simulink subsystem "drive"  (R2022a)
settings: Solver=VariableStepAuto  StartTime=0.0  StopTime=10.0  RelTol=1e-3
settings Model: Creator=12191  LastModifiedBy=12191

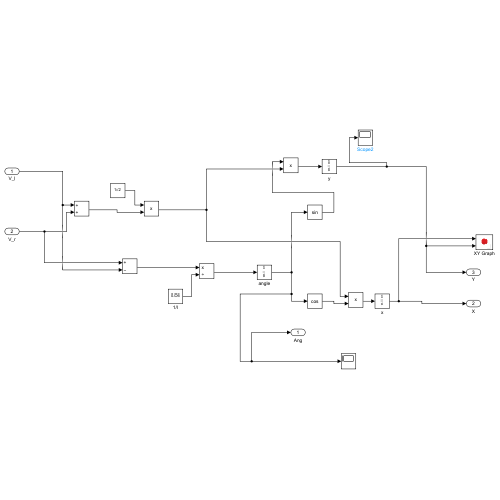
[thumbnail: Simulink's stored preview of the top-level diagram]
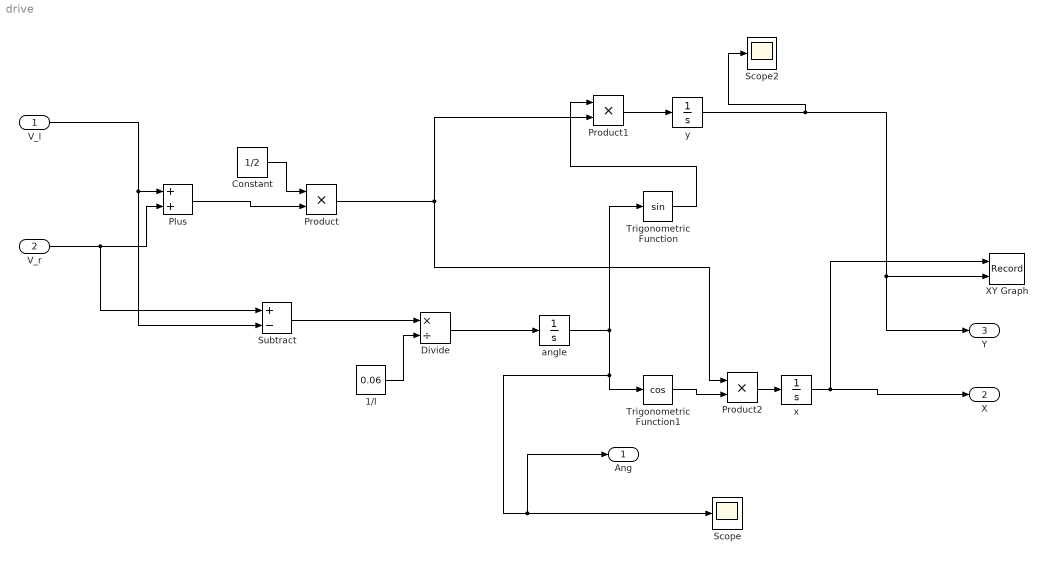
== system drive ==
  V_l : Inport
  V_r : Inport  Port=2
  1/l : Constant  Value=0.06
  Constant : Constant  Value=1/2
  Divide : Product  Inputs=*/
  Plus : Sum
  Product : Product
  Product1 : Product
  Product2 : Product
  Scope : Scope
  Scope2 : Scope
  Subtract : Sum  Inputs=+-
  Trigonometric Function : Trigonometry
  Trigonometric Function1 : Trigonometry  Operator=cos
  XY Graph : Record  FileSettingsInternal="{\"entries\":[{\"content\":{\"excelSettings\":{\"content\":{},\"type\":\"Streamout.ExcelSettings\"}},\"type\":\"Streamout.FileSettingStorage\",\"uuid\":\"175092fb-4bae-40dd-9490-6dec79859699\"}],\"packageUris\":[\"http://schema.mathworks.com/mf0/streamout_blocks/R2020a\"],\"version\":\"1.0\"}"  Layout=[1 1]  SignalsInternal="{\"entries\":[{\"content\":{\"signals\":[{\"content\":{\"blockPath\":[\"drive/XY Graph\"],\"channel\":[],\"dimensions\":[1],\"domain\":\"drive/XY Graph\",\"lineColor\":\"#a2142f\",\"plots\":[],\"port\":1,\"sid\":[],\"signalID\":747,\"signalName\":\"angle2\"},\"type\":\"RecordBlkView.Signal\",\"uuid\":\"ca3ea469-2ea0-4ac0-a534-a51894ec1fa5\"},{\"content\":{\"blockPath\":[\"drive/XY Graph\"],\"channel\":[],\"dimensions\":[1],\"domain\":\"drive/XY Graph\",\"lineColor\":\"#139fff\",\"plots\":[],\"port\":2,\"sid\":[],\"signalID\":750,\"signalName\":\"angle1\"},\"type\":\"RecordBlkView.Signal\",\"uuid\":\"6b707983-fc52-4215-b12b-d22f56800b9f\"}]},\"type\":\"RecordBlkView.InputSignals\",\"uuid\":\"37fc4046-acd5-4136-a23c-9627ac4b1407\"}],\"packageUris\":[\"http://schema.mathworks.com/mf0/streamout_blocks/R2020a\"],\"version\":\"1.0\"}"  VisualizationBindings="{\"sparklinesplugin\":{\"info\":[{\"bindingParametersList\":[],\"subplotID\":1}]}}"  CompatibilityTag=XY
  angle : Integrator
  x : Integrator
  y : Integrator
  Ang : Outport
  X : Outport  Port=2
  Y : Outport  Port=3
  wires:
  Subtract/1 -> Divide/1
  Constant/1 -> Product/1
  Divide/1 -> angle/1
  Trigonometric Function1/1 -> Product2/2
  V_r/1 -> Subtract/1, Plus/2
  1/l/1 -> Divide/2
  angle/1 -> Trigonometric Function1/1, Ang/1, Scope/1, Trigonometric Function/1
  V_l/1 -> Subtract/2, Plus/1
  Trigonometric Function/1 -> Product1/1
  Product1/1 -> y/1
  Product2/1 -> x/1
  y/1 -> Scope2/1, Y/1, XY Graph/2
  Product/1 -> Product1/2, Product2/1
  Plus/1 -> Product/2
  x/1 -> X/1, XY Graph/1
